simulink model "Model_Direct_design_controller_SS_nominal_tracking_system"  (R2024b)
settings: Solver=VariableStepDiscrete  StartTime=0.0  StopTime=3  RelTol=1e-3
values from neighbouring files (symbols this model uses):
  Ts = Ts_values(i)    [A_final_results.m]
undefined symbols (not defined in the file or in its folder): sigmaD_tf_den, sigmaD_tf_num
settings Model: Creator=Riccardo Grosso  LastModifiedBy=Buton

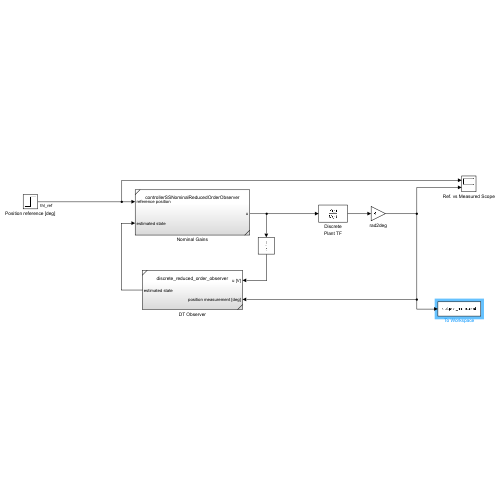
[thumbnail: Simulink's stored preview of the top-level diagram]
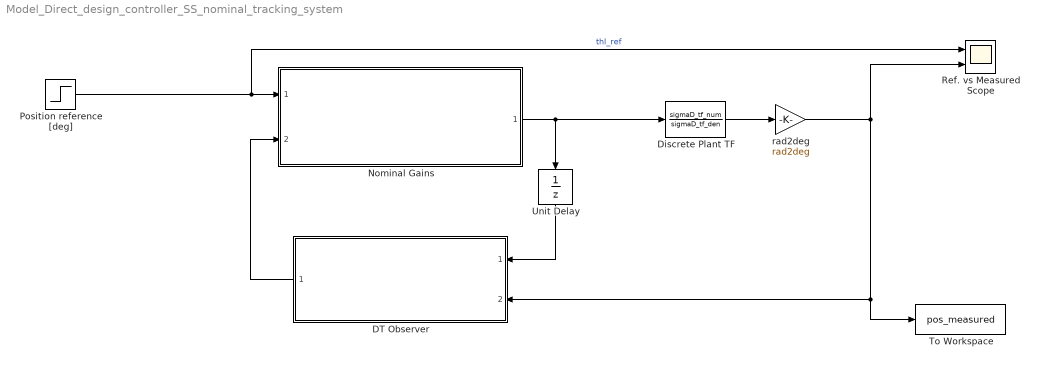
== system Model_Direct_design_controller_SS_nominal_tracking_system ==
  DT Observer : Subsystem  ReferencedSubsystem=discrete_reduced_order_observer
  Discrete Plant TF : DiscreteTransferFcn  Numerator=sigmaD_tf_num  Denominator=sigmaD_tf_den
  Nominal Gains : Subsystem  ReferencedSubsystem=controllerSSNominalReducedOrderObserver
  Position reference [deg] : Step  Time=0  After=50  SampleTime=Ts
  Ref. vs Measured Scope : Scope  NumInputPorts=2
  To Workspace : ToWorkspace  VariableName=pos_measured  SaveFormat=Timeseries  SampleTime=-1
  Unit Delay : UnitDelay  SampleTime=-1  HasFrameUpgradeWarning=on
  rad2deg : Gain  Gain=rad2deg
  wires:
  Position reference [deg]/1 -> Ref. vs Measured Scope/1, Nominal Gains/1  "thl_ref"
  Nominal Gains/1 -> Discrete Plant TF/1, Unit Delay/1
  DT Observer/1 -> Nominal Gains/2
  Discrete Plant TF/1 -> rad2deg/1
  rad2deg/1 -> To Workspace/1, DT Observer/2, Ref. vs Measured Scope/2
  Unit Delay/1 -> DT Observer/1
